simulink library "inp"  (R2021b)
settings: Solver=VariableStepAuto  StartTime=0.0  StopTime=10.0  RelTol=1e-3
undefined symbols (not defined in the file): C_TASK_5MS_S, FALSE, KINP_AcoreReadyToSlp_flg_ovrdflg, KINP_AcoreReadyToSlp_flg_ovrdval, KINP_AllowMovThd_OTA_enum_ovrdflg, KINP_AllowMovThd_OTA_enum_ovrdval, KINP_APSAngleTarget_Deg_ovrdflg, KINP_APSAngleTarget_Deg_ovrdval, KINP_APSDecReq_mps2_ovrdflg, KINP_APSDecReq_mps2_ovrdval, KINP_APSDecReqA_flg_ovrdflg, KINP_APSDecReqA_flg_ovrdval, KINP_APSDFLL_cm_ovrdflg, KINP_APSDFLL_cm_ovrdval, KINP_APSDFLR_cm_ovrdflg, KINP_APSDFLR_cm_ovrdval, KINP_APSDRLL_cm_ovrdflg, KINP_APSDRLL_cm_ovrdval, KINP_APSDRLR_cm_ovrdflg, KINP_APSDRLR_cm_ovrdval, KINP_APSExitCondition_enum_ovrdflg, KINP_APSExitCondition_enum_ovrdval, KINP_APSHWVer_enum_ovrdflg, KINP_APSHWVer_enum_ovrdval, KINP_APSProgressPCT_pct_ovrdflg, KINP_APSProgressPCT_pct_ovrdval, KINP_APSPwrReq_enum_ovrdflg, KINP_APSPwrReq_enum_ovrdval, KINP_APSReq_enum_ovrdflg, KINP_APSReq_enum_ovrdval, KINP_APSRQDisplay_enum_ovrdflg, KINP_APSRQDisplay_enum_ovrdval, KINP_APSRqEPASCtrl_flg_ovrdflg, KINP_APSRqEPASCtrl_flg_ovrdval, KINP_APSShiftPosnReq_enum_ovrdval, KINP_APSShiftPosnReq_enum_ovrflg, KINP_APSSpeedCMD_kph_ovrdval, KINP_APSSpeedCMD_kph_ovrflg, KINP_APSStaSystem_enum_ovrdflg, KINP_APSStaSystem_enum_ovrdval, KINP_APSSWVer_enum_ovrdflg, KINP_APSSWVer_enum_ovrdval, KINP_APSVMCReqA_flg_ovrdval, KINP_APSVMCReqA_flg_ovrflg, KINP_APSVRqEPASCtrl_flg_ovrdflg, KINP_APSVRqEPASCtrl_flg_ovrdval, KINP_AuxBattVolmV_mV_ovrdflg, KINP_AuxBattVolmV_mV_ovrdval, KINP_CAASSta_enum_ovrdflg, KINP_CAASSta_enum_ovrdval, KINP_CAASVMCReqA_flg_ovrdval, KINP_CAASVMCReqA_flg_ovrflg, KINP_CAN1BusOff_flg_ovrdflg, KINP_CAN1BusOff_flg_ovrdval, KINP_CAN2BusOff_flg_ovrdflg, KINP_CAN2BusOff_flg_ovrdval, KINP_CAN3BusOff_flg_ovrdflg, KINP_CAN3BusOff_flg_ovrdval, KINP_CAN4BusOff_flg_ovrdflg, KINP_CAN4BusOff_flg_ovrdval ... (+152)
libraries: FVT_lib x1037, hcu_lib x1
(part 6 of 34)

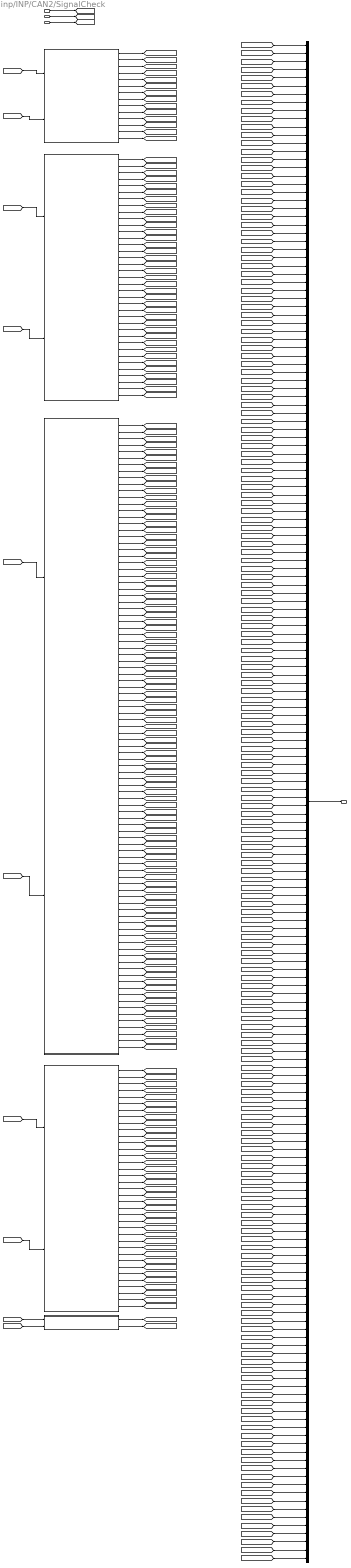
== system inp/INP/CAN2/SignalCheck ==
  inp_CanValid_bus : Inport
  TASK_TIME_S : Inport  Port=2
  BHAL_outputs : Inport  Port=3
  HMI1 : Subsystem
  IVI1 : Subsystem
  IVI2 : Subsystem
  IVI3 : Subsystem
  METER1 : Subsystem
  bus_creator : BusCreator  Inputs=186
  inp_Hal_bus : Outport
  wires:
  inp_CanValid_bus/1 -> [inp_CanValid_bus]
  TASK_TIME_S/1 -> [TASK_TIME_S]
  BHAL_outputs/1 -> [BHAL_outputs]
  [BHAL_outputs] -> HMI1/1(BHAL_outputs)
  [inp_CanValid_bus] -> HMI1/2(inp_CanValid_bus)
  HMI1/1(VINP_HMIACAirIntMCmd_flg) -> [VINP_HMIACAirIntMCmd_flg]
  HMI1/2(VINP_HMIACAirIntPCmd_flg) -> [VINP_HMIACAirIntPCmd_flg]
  HMI1/3(VINP_HMIACAutoBtnCmd_flg) -> [VINP_HMIACAutoBtnCmd_flg]
  HMI1/4(VINP_HMIACBtnCmd_flg) -> [VINP_HMIACBtnCmd_flg]
  HMI1/5(VINP_HMIACFrDefogBtnCmd_flg) -> [VINP_HMIACFrDefogBtnCmd_flg]
  HMI1/6(VINP_HMIACRecycleBtnCmd_flg) -> [VINP_HMIACRecycleBtnCmd_flg]
  HMI1/7(VINP_HMIACWindDirMCmd_flg) -> [VINP_HMIACWindDirMCmd_flg]
  HMI1/8(VINP_HMIACWindDirPCmd_flg) -> [VINP_HMIACWindDirPCmd_flg]
  HMI1/9(VINP_HMIAutoInterLightCmd_flg) -> [VINP_HMIAutoInterLightCmd_flg]
  HMI1/10(VINP_HMIBCMPostDefogBtnCmd_flg) -> [VINP_HMIBCMPostDefogBtnCmd_flg]
  HMI1/11(VINP_HMIZ1SetTMCmd_flg) -> [VINP_HMIZ1SetTMCmd_flg]
  HMI1/12(VINP_HMIZ1SetTPCmd_flg) -> [VINP_HMIZ1SetTPCmd_flg]
  HMI1/13(VINP_HMIZ2SetTMCmd_flg) -> [VINP_HMIZ2SetTMCmd_flg]
  HMI1/14(VINP_HMIZ2SetTPCmd_flg) -> [VINP_HMIZ2SetTPCmd_flg]
  [BHAL_outputs] -> IVI1/1(BHAL_outputs)
  [inp_CanValid_bus] -> IVI1/2(inp_CanValid_bus)
  IVI1/1(VINP_AmbLighLowBatAlertSW_flg) -> [VINP_AmbLighLowBatAlertSW_flg]
  IVI1/2(VINP_AmbLighSafetyAlertSW_flg) -> [VINP_AmbLighSafetyAlertSW_flg]
  IVI1/3(VINP_AmbLightBrightnessSet_enum) -> [VINP_AmbLightBrightnessSet_enum]
  IVI1/4(VINP_AmbLightColorSet_enum) -> [VINP_AmbLightColorSet_enum]
  IVI1/5(VINP_AmbLightDimInDarkSW_flg) -> [VINP_AmbLightDimInDarkSW_flg]
  IVI1/6(VINP_AmbLightSW_flg) -> [VINP_AmbLightSW_flg]
  IVI1/7(VINP_AmbLightWlcmLightSW_flg) -> [VINP_AmbLightWlcmLightSW_flg]
  IVI1/8(VINP_FCPFrEvtBtnACMaxReq_flg) -> [VINP_FCPFrEvtBtnACMaxReq_flg]
  IVI1/9(VINP_FCPFrEvtBtnACReq_flg) -> [VINP_FCPFrEvtBtnACReq_flg]
  IVI1/10(VINP_FCPFrEvtBtnAutoReq_flg) -> [VINP_FCPFrEvtBtnAutoReq_flg]
  IVI1/11(VINP_FCPFrEvtBtnSyncReq_flg) -> [VINP_FCPFrEvtBtnSyncReq_flg]
  IVI1/12(VINP_IVIAutoWipHSpdSWCmd_flg) -> [VINP_IVIAutoWipHSpdSWCmd_flg]
  IVI1/13(VINP_IVICreateAccReqSta_enum) -> [VINP_IVICreateAccReqSta_enum]
  IVI1/14(VINP_IVIDelAccReqSta_enum) -> [VINP_IVIDelAccReqSta_enum]
  IVI1/15(VINP_IVIDrivingLockSWSta_flg) -> [VINP_IVIDrivingLockSWSta_flg]
  IVI1/16(VINP_IVIFrTrunkUnlockReqSta_flg) -> [VINP_IVIFrTrunkUnlockReqSta_flg]
  IVI1/17(VINP_IVILinkAccReqSta_flg) -> [VINP_IVILinkAccReqSta_flg]
  IVI1/18(VINP_IVILinkAccSta_enum) -> [VINP_IVILinkAccSta_enum]
  IVI1/19(VINP_IVILinkKeySta_enum) -> [VINP_IVILinkKeySta_enum]
  IVI1/20(VINP_IVILocatedSTA_enum) -> [VINP_IVILocatedSTA_enum]
  IVI1/21(VINP_IVILockSoundSWSta_flg) -> [VINP_IVILockSoundSWSta_flg]
  IVI1/22(VINP_IVISWCVibModeSta_enum) -> [VINP_IVISWCVibModeSta_enum]
  IVI1/23(VINP_IVIStoppingUnlockSWSta_flg) -> [VINP_IVIStoppingUnlockSWSta_flg]
  IVI1/24(VINP_IVITimeCheck_enum) -> [VINP_IVITimeCheck_enum]
  IVI1/25(VINP_IVITimeDay_DAY) -> [VINP_IVITimeDay_DAY]
  IVI1/26(VINP_IVITimeHour_hr) -> [VINP_IVITimeHour_hr]
  IVI1/27(VINP_IVITimeMinute_min) -> [VINP_IVITimeMinute_min]
  IVI1/28(VINP_IVITimeMonth_MONTH) -> [VINP_IVITimeMonth_MONTH]
  IVI1/29(VINP_IVITimeSecond_s) -> [VINP_IVITimeSecond_s]
  IVI1/30(VINP_IVITimeYear_YEAR) -> [VINP_IVITimeYear_YEAR]
  IVI1/31(VINP_IVIWPTCSWSta_flg) -> [VINP_IVIWPTCSWSta_flg]
  IVI1/32(VINP_IVIsigScreenReqSta_flg) -> [VINP_IVIsigScreenReqSta_flg]
  IVI1/33(VINP_LINKtoDrive_flg) -> [VINP_LINKtoDrive_flg]
  IVI1/34(VINP_OpenDrOpenWdoSW_flg) -> [VINP_OpenDrOpenWdoSW_flg]
  IVI1/35(VINP_PWCONTINUEUSE_flg) -> [VINP_PWCONTINUEUSE_flg]
  IVI1/36(VINP_SmartEcoModeSW_flg) -> [VINP_SmartEcoModeSW_flg]
  IVI1/37(VINP_UserSet_enum) -> [VINP_UserSet_enum]
  [BHAL_outputs] -> IVI2/1(BHAL_outputs)
  [inp_CanValid_bus] -> IVI2/2(inp_CanValid_bus)
  IVI2/1(VINP_ACChgCurSet_A) -> [VINP_ACChgCurSet_A]
  IVI2/2(VINP_AVMErrSTA_flg) -> [VINP_AVMErrSTA_flg]
  IVI2/3(VINP_AVMOFFRecButt_flg) -> [VINP_AVMOFFRecButt_flg]
  IVI2/4(VINP_AVMParkingmode_enum) -> [VINP_AVMParkingmode_enum]
  IVI2/5(VINP_AVMparkingcancel_enum) -> [VINP_AVMparkingcancel_enum]
  IVI2/6(VINP_AVMparkingexcute_enum) -> [VINP_AVMparkingexcute_enum]
  IVI2/7(VINP_ApproachUnlockSW_flg) -> [VINP_ApproachUnlockSW_flg]
  IVI2/8(VINP_CAASSw_enum) -> [VINP_CAASSw_enum]
  IVI2/9(VINP_CDLLockButt_flg) -> [VINP_CDLLockButt_flg]
  IVI2/10(VINP_CDLUnlockButt_flg) -> [VINP_CDLUnlockButt_flg]
  IVI2/11(VINP_DSEATantiset_flg) -> [VINP_DSEATantiset_flg]
  IVI2/12(VINP_DSEATentryfunset_flg) -> [VINP_DSEATentryfunset_flg]
  IVI2/13(VINP_DSEATventreq_enum) -> [VINP_DSEATventreq_enum]
  IVI2/14(VINP_Distanceunit_flg) -> [VINP_Distanceunit_flg]
  IVI2/15(VINP_ESCSWCmd_enum) -> [VINP_ESCSWCmd_enum]
  IVI2/16(VINP_FSOffSw_enum) -> [VINP_FSOffSw_enum]
  IVI2/17(VINP_FollowMeSW_flg) -> [VINP_FollowMeSW_flg]
  IVI2/18(VINP_GPSLAT_s) -> [VINP_GPSLAT_s]
  IVI2/19(VINP_GPSLONG_enum) -> [VINP_GPSLONG_enum]
  IVI2/20(VINP_HeadLampSW_enum) -> [VINP_HeadLampSW_enum]
  IVI2/21(VINP_HoodLatchSW_enum) -> [VINP_HoodLatchSW_enum]
  IVI2/22(VINP_IVIACCAdaptiveSta_flg) -> [VINP_IVIACCAdaptiveSta_flg]
  IVI2/23(VINP_IVIAirIntZ3Cmd_enum) -> [VINP_IVIAirIntZ3Cmd_enum]
  IVI2/24(VINP_IVIChargePortSWSta_flg) -> [VINP_IVIChargePortSWSta_flg]
  IVI2/25(VINP_IVICreepSWReq_flg) -> [VINP_IVICreepSWReq_flg]
  IVI2/26(VINP_IVIDSEATHeaterCmd_enum) -> [VINP_IVIDSEATHeaterCmd_enum]
  IVI2/27(VINP_IVIDSEATFroEdgeHeightCmd_enum) -> [VINP_IVIDSEATFroEdgeHeightCmd_enum]
  IVI2/28(VINP_IVIDSEATHeightCmd_enum) -> [VINP_IVIDSEATHeightCmd_enum]
  IVI2/29(VINP_IVIDSEATMemory1Sta_flg) -> [VINP_IVIDSEATMemory1Sta_flg]
  IVI2/30(VINP_IVIDSEATMemory2Sta_flg) -> [VINP_IVIDSEATMemory2Sta_flg]
  IVI2/31(VINP_IVIDSEATMemoryOPTCLSSta_flg) -> [VINP_IVIDSEATMemoryOPTCLSSta_flg]
  IVI2/32(VINP_IVIDSEATReclineCmd_enum) -> [VINP_IVIDSEATReclineCmd_enum]
  IVI2/33(VINP_IVIDSEATSlideCmd_enum) -> [VINP_IVIDSEATSlideCmd_enum]
  IVI2/34(VINP_IVIFGSAirIntCmd_enum) -> [VINP_IVIFGSAirIntCmd_enum]
  IVI2/35(VINP_IVIFGSChCmd_enum) -> [VINP_IVIFGSChCmd_enum]
  IVI2/36(VINP_IVIIONSWCmd_flg) -> [VINP_IVIIONSWCmd_flg]
  IVI2/37(VINP_IVIISAOffsetSpd_enum) -> [VINP_IVIISAOffsetSpd_enum]
  IVI2/38(VINP_IVINightModeSta_flg) -> [VINP_IVINightModeSta_flg]
  IVI2/39(VINP_IVIPSEATHeaterCmd_enum) -> [VINP_IVIPSEATHeaterCmd_enum]
  IVI2/40(VINP_IVIPSEATReclineCmd_enum) -> [VINP_IVIPSEATReclineCmd_enum]
  IVI2/41(VINP_IVIPSEATSlideCmd_enum) -> [VINP_IVIPSEATSlideCmd_enum]
  IVI2/42(VINP_IVIPTGModeSW_enum) -> [VINP_IVIPTGModeSW_enum]
  IVI2/43(VINP_IVIPTGOpenHeight_enum) -> [VINP_IVIPTGOpenHeight_enum]
  IVI2/44(VINP_IVIPTGStaSW_enum) -> [VINP_IVIPTGStaSW_enum]
  IVI2/45(VINP_IVIPTGUSStaSW_flg) -> [VINP_IVIPTGUSStaSW_flg]
  IVI2/46(VINP_IVIPWModeReq_enum) -> [VINP_IVIPWModeReq_enum]
  IVI2/47(VINP_IVIPwrLockSW_enum) -> [VINP_IVIPwrLockSW_enum]
  IVI2/48(VINP_IVIPwroffreq_flg) -> [VINP_IVIPwroffreq_flg]
  IVI2/49(VINP_IVIRRDefReq_flg) -> [VINP_IVIRRDefReq_flg]
  IVI2/50(VINP_IVIReqV2L_enum) -> [VINP_IVIReqV2L_enum]
  IVI2/51(VINP_IVISWCRUndefinedSta_enum) -> [VINP_IVISWCRUndefinedSta_enum]
  IVI2/52(VINP_IVIScreen_enum) -> [VINP_IVIScreen_enum]
  IVI2/53(VINP_IVIStartChgreq_flg) -> [VINP_IVIStartChgreq_flg]
  IVI2/54(VINP_IVIStatus_flg) -> [VINP_IVIStatus_flg]
  IVI2/55(VINP_IVIStopChgreq_flg) -> [VINP_IVIStopChgreq_flg]
  IVI2/56(VINP_IVITrailerCheckReqSta_flg) -> [VINP_IVITrailerCheckReqSta_flg]
  IVI2/57(VINP_IVITrailerModeSWSta_flg) -> [VINP_IVITrailerModeSWSta_flg]
  IVI2/58(VINP_IVITriggerreq_flg) -> [VINP_IVITriggerreq_flg]
  IVI2/59(VINP_IVIUnlockChgreq_flg) -> [VINP_IVIUnlockChgreq_flg]
  IVI2/60(VINP_IVIWIMAINSW_flg) -> [VINP_IVIWIMAINSW_flg]
  IVI2/61(VINP_LDrvControlCommand_pct) -> [VINP_LDrvControlCommand_pct]
  IVI2/62(VINP_LPasControlCommand_pct) -> [VINP_LPasControlCommand_pct]
  IVI2/63(VINP_LRLDControlCommand_pct) -> [VINP_LRLDControlCommand_pct]
  IVI2/64(VINP_LRRDControlCommand_pct) -> [VINP_LRRDControlCommand_pct]
  IVI2/65(VINP_LightShowStartReq_flg) -> [VINP_LightShowStartReq_flg]
  IVI2/66(VINP_LightShowStopReq_flg) -> [VINP_LightShowStopReq_flg]
  IVI2/67(VINP_MFRDNBrightReq_pct) -> [VINP_MFRDNBrightReq_pct]
  IVI2/68(VINP_OFFACMODE_enum) -> [VINP_OFFACMODE_enum]
  IVI2/69(VINP_PSEATventreq_enum) -> [VINP_PSEATventreq_enum]
  IVI2/70(VINP_PerdV2L_enum) -> [VINP_PerdV2L_enum]
  IVI2/71(VINP_RFogLampSW_flg) -> [VINP_RFogLampSW_flg]
  IVI2/72(VINP_RollModeSWCmd_enum) -> [VINP_RollModeSWCmd_enum]
  IVI2/73(VINP_RoomLampMode_flg) -> [VINP_RoomLampMode_flg]
  IVI2/74(VINP_SOCADJBUTT_flg) -> [VINP_SOCADJBUTT_flg]
  IVI2/75(VINP_SOCLimitSet_pct) -> [VINP_SOCLimitSet_pct]
  IVI2/76(VINP_SOCV2LLimit_pct) -> [VINP_SOCV2LLimit_pct]
  IVI2/77(VINP_SchedChgStart_flg) -> [VINP_SchedChgStart_flg]
  IVI2/78(VINP_SchedChgStop_flg) -> [VINP_SchedChgStop_flg]
  IVI2/79(VINP_SchedChgbutt_flg) -> [VINP_SchedChgbutt_flg]
  IVI2/80(VINP_SchedChglimit_pct) -> [VINP_SchedChglimit_pct]
  IVI2/81(VINP_SchedChgwake_flg) -> [VINP_SchedChgwake_flg]
  IVI2/82(VINP_SenstivityPosition_enum) -> [VINP_SenstivityPosition_enum]
  IVI2/83(VINP_SetUnlockSingle_flg) -> [VINP_SetUnlockSingle_flg]
  IVI2/84(VINP_TCSSWCmd_enum) -> [VINP_TCSSWCmd_enum]
  IVI2/85(VINP_TPMSCaliButt_flg) -> [VINP_TPMSCaliButt_flg]
  IVI2/86(VINP_TPMSResButt_flg) -> [VINP_TPMSResButt_flg]
  IVI2/87(VINP_TurnSwTimeSet_enum) -> [VINP_TurnSwTimeSet_enum]
  IVI2/88(VINP_WalkawayLockSW_flg) -> [VINP_WalkawayLockSW_flg]
  IVI2/89(VINP_WlcmLightMode_enum) -> [VINP_WlcmLightMode_enum]
  IVI2/90(VINP_sigAirIntenZon1Req_enum) -> [VINP_sigAirIntenZon1Req_enum]
  IVI2/91(VINP_sigDfrstReq_flg) -> [VINP_sigDfrstReq_flg]
  IVI2/92(VINP_sigFaceReq_flg) -> [VINP_sigFaceReq_flg]
  IVI2/93(VINP_sigFootReq_flg) -> [VINP_sigFootReq_flg]
  IVI2/94(VINP_sigRecircReq_flg) -> [VINP_sigRecircReq_flg]
  IVI2/95(VINP_sigSetTempZon1Req_C) -> [VINP_sigSetTempZon1Req_C]
  IVI2/96(VINP_sigSetTempZon2Req_C) -> [VINP_sigSetTempZon2Req_C]
  [BHAL_outputs] -> IVI3/1(BHAL_outputs)
  [inp_CanValid_bus] -> IVI3/2(inp_CanValid_bus)
  IVI3/1(VINP_IVICLBlowerYSta_pct) -> [VINP_IVICLBlowerYSta_pct]
  IVI3/2(VINP_IVICLBlowerZSta_pct) -> [VINP_IVICLBlowerZSta_pct]
  IVI3/3(VINP_IVICRBlowerYSta_pct) -> [VINP_IVICRBlowerYSta_pct]
  IVI3/4(VINP_IVICRBlowerZSta_pct) -> [VINP_IVICRBlowerZSta_pct]
  IVI3/5(VINP_IVIDrBlowerModeSta_enum) -> [VINP_IVIDrBlowerModeSta_enum]
  IVI3/6(VINP_IVIDrBlowerYSta_pct) -> [VINP_IVIDrBlowerYSta_pct]
  IVI3/7(VINP_IVIDrBlowerZSta_pct) -> [VINP_IVIDrBlowerZSta_pct]
  IVI3/8(VINP_IVIHMICustmiFunSta_enum) -> [VINP_IVIHMICustmiFunSta_enum]
  IVI3/9(VINP_IVIHMICustmiKEYSta_enum) -> [VINP_IVIHMICustmiKEYSta_enum]
  IVI3/10(VINP_IVILSEATventCmd_enum) -> [VINP_IVILSEATventCmd_enum]
  IVI3/11(VINP_IVIMLFMostCmd_flg) -> [VINP_IVIMLFMostCmd_flg]
  IVI3/12(VINP_IVIMLFootLiftCmd_enum) -> [VINP_IVIMLFootLiftCmd_enum]
  IVI3/13(VINP_IVIMLNapModeCmd_flg) -> [VINP_IVIMLNapModeCmd_flg]
  IVI3/14(VINP_IVIMLReclinerCmd_enum) -> [VINP_IVIMLReclinerCmd_enum]
  IVI3/15(VINP_IVIMLRestoreCmd_flg) -> [VINP_IVIMLRestoreCmd_flg]
  IVI3/16(VINP_IVIMLSEATventCmd_enum) -> [VINP_IVIMLSEATventCmd_enum]
  IVI3/17(VINP_IVIMLSeatLiftCmd_enum) -> [VINP_IVIMLSeatLiftCmd_enum]
  IVI3/18(VINP_IVIMLSldRestoreCmd_flg) -> [VINP_IVIMLSldRestoreCmd_flg]
  IVI3/19(VINP_IVIMLSliderCmd_enum) -> [VINP_IVIMLSliderCmd_enum]
  IVI3/20(VINP_IVIMLZeroGravityCmd_flg) -> [VINP_IVIMLZeroGravityCmd_flg]
  IVI3/21(VINP_IVIMRFMostCmd_flg) -> [VINP_IVIMRFMostCmd_flg]
  IVI3/22(VINP_IVIMRFootLiftCmd_enum) -> [VINP_IVIMRFootLiftCmd_enum]
  IVI3/23(VINP_IVIMRNapModeCmd_flg) -> [VINP_IVIMRNapModeCmd_flg]
  IVI3/24(VINP_IVIMRReclinerCmd_enum) -> [VINP_IVIMRReclinerCmd_enum]
  IVI3/25(VINP_IVIMRRestoreCmd_flg) -> [VINP_IVIMRRestoreCmd_flg]
  IVI3/26(VINP_IVIMRSEATventCmd_enum) -> [VINP_IVIMRSEATventCmd_enum]
  IVI3/27(VINP_IVIMRSeatLiftCmd_enum) -> [VINP_IVIMRSeatLiftCmd_enum]
  IVI3/28(VINP_IVIMRSldRestoreCmd_flg) -> [VINP_IVIMRSldRestoreCmd_flg]
  IVI3/29(VINP_IVIMRSliderCmd_enum) -> [VINP_IVIMRSliderCmd_enum]
  IVI3/30(VINP_IVIMRZeroGravityCmd_flg) -> [VINP_IVIMRZeroGravityCmd_flg]
  IVI3/31(VINP_IVIPsBlowerModeSta_enum) -> [VINP_IVIPsBlowerModeSta_enum]
  IVI3/32(VINP_IVIPsBlowerYSta_pct) -> [VINP_IVIPsBlowerYSta_pct]
  IVI3/33(VINP_IVIPsBlowerZSta_pct) -> [VINP_IVIPsBlowerZSta_pct]
  IVI3/34(VINP_IVIRSEATventCmd_enum) -> [VINP_IVIRSEATventCmd_enum]
  IVI3/35(VINP_IVISnowModeCmd_flg) -> [VINP_IVISnowModeCmd_flg]
  IVI3/36(VINP_IVIUserTakeOverAPSSta_flg) -> [VINP_IVIUserTakeOverAPSSta_flg]
  IVI3/37(VINP_IVIZon1WindDirSWReqSta_flg) -> [VINP_IVIZon1WindDirSWReqSta_flg]
  [BHAL_outputs] -> METER1/1(BHAL_outputs)
  [inp_CanValid_bus] -> METER1/2(inp_CanValid_bus)
  METER1/1(VINP_METERKPHCalcu_kph) -> [VINP_METERKPHCalcu_kph]
  METER1/2(VINP_ODOMETER_km) -> [VINP_ODOMETER_km]
  bus_creator/1 -> inp_Hal_bus/1
  [VINP_HMIACAirIntMCmd_flg] -> bus_creator/1
  [VINP_HMIACAirIntPCmd_flg] -> bus_creator/2
  [VINP_HMIACAutoBtnCmd_flg] -> bus_creator/3
  [VINP_HMIACBtnCmd_flg] -> bus_creator/4
  [VINP_HMIACFrDefogBtnCmd_flg] -> bus_creator/5
  [VINP_HMIACRecycleBtnCmd_flg] -> bus_creator/6
  [VINP_HMIACWindDirMCmd_flg] -> bus_creator/7
  [VINP_HMIACWindDirPCmd_flg] -> bus_creator/8
  [VINP_HMIAutoInterLightCmd_flg] -> bus_creator/9
  [VINP_HMIBCMPostDefogBtnCmd_flg] -> bus_creator/10
  [VINP_HMIZ1SetTMCmd_flg] -> bus_creator/11
  [VINP_HMIZ1SetTPCmd_flg] -> bus_creator/12
  [VINP_HMIZ2SetTMCmd_flg] -> bus_creator/13
  [VINP_HMIZ2SetTPCmd_flg] -> bus_creator/14
  [VINP_AmbLighLowBatAlertSW_flg] -> bus_creator/15
  [VINP_AmbLighSafetyAlertSW_flg] -> bus_creator/16
  [VINP_AmbLightBrightnessSet_enum] -> bus_creator/17
  [VINP_AmbLightColorSet_enum] -> bus_creator/18
  [VINP_AmbLightDimInDarkSW_flg] -> bus_creator/19
  [VINP_AmbLightSW_flg] -> bus_creator/20
  [VINP_AmbLightWlcmLightSW_flg] -> bus_creator/21
  [VINP_FCPFrEvtBtnACMaxReq_flg] -> bus_creator/22
  [VINP_FCPFrEvtBtnACReq_flg] -> bus_creator/23
  [VINP_FCPFrEvtBtnAutoReq_flg] -> bus_creator/24
  [VINP_FCPFrEvtBtnSyncReq_flg] -> bus_creator/25
  [VINP_IVIAutoWipHSpdSWCmd_flg] -> bus_creator/26
  [VINP_IVICreateAccReqSta_enum] -> bus_creator/27
  [VINP_IVIDelAccReqSta_enum] -> bus_creator/28
  [VINP_IVIDrivingLockSWSta_flg] -> bus_creator/29
  [VINP_IVIFrTrunkUnlockReqSta_flg] -> bus_creator/30
  [VINP_IVILinkAccReqSta_flg] -> bus_creator/31
  [VINP_IVILinkAccSta_enum] -> bus_creator/32
  [VINP_IVILinkKeySta_enum] -> bus_creator/33
  [VINP_IVILocatedSTA_enum] -> bus_creator/34
  [VINP_IVILockSoundSWSta_flg] -> bus_creator/35
  [VINP_IVISWCVibModeSta_enum] -> bus_creator/36
  [VINP_IVIStoppingUnlockSWSta_flg] -> bus_creator/37
  [VINP_IVITimeCheck_enum] -> bus_creator/38
  [VINP_IVITimeDay_DAY] -> bus_creator/39
  [VINP_IVITimeHour_hr] -> bus_creator/40
  [VINP_IVITimeMinute_min] -> bus_creator/41
  [VINP_IVITimeMonth_MONTH] -> bus_creator/42
  [VINP_IVITimeSecond_s] -> bus_creator/43
  [VINP_IVITimeYear_YEAR] -> bus_creator/44
  [VINP_IVIWPTCSWSta_flg] -> bus_creator/45
  [VINP_IVIsigScreenReqSta_flg] -> bus_creator/46
  [VINP_LINKtoDrive_flg] -> bus_creator/47
  [VINP_OpenDrOpenWdoSW_flg] -> bus_creator/48
  [VINP_PWCONTINUEUSE_flg] -> bus_creator/49
  [VINP_SmartEcoModeSW_flg] -> bus_creator/50
  [VINP_UserSet_enum] -> bus_creator/51
  [VINP_ACChgCurSet_A] -> bus_creator/52
  [VINP_AVMErrSTA_flg] -> bus_creator/53
  [VINP_AVMOFFRecButt_flg] -> bus_creator/54
  [VINP_AVMParkingmode_enum] -> bus_creator/55
  [VINP_AVMparkingcancel_enum] -> bus_creator/56
  [VINP_AVMparkingexcute_enum] -> bus_creator/57
  [VINP_ApproachUnlockSW_flg] -> bus_creator/58
  [VINP_CAASSw_enum] -> bus_creator/59
  [VINP_CDLLockButt_flg] -> bus_creator/60
  [VINP_CDLUnlockButt_flg] -> bus_creator/61
  [VINP_DSEATantiset_flg] -> bus_creator/62
  [VINP_DSEATentryfunset_flg] -> bus_creator/63
  [VINP_DSEATventreq_enum] -> bus_creator/64
  [VINP_Distanceunit_flg] -> bus_creator/65
  [VINP_ESCSWCmd_enum] -> bus_creator/66
  [VINP_FSOffSw_enum] -> bus_creator/67
  [VINP_FollowMeSW_flg] -> bus_creator/68
  [VINP_GPSLAT_s] -> bus_creator/69
  [VINP_GPSLONG_enum] -> bus_creator/70
  [VINP_HeadLampSW_enum] -> bus_creator/71
  [VINP_HoodLatchSW_enum] -> bus_creator/72
  [VINP_IVIACCAdaptiveSta_flg] -> bus_creator/73
  [VINP_IVIAirIntZ3Cmd_enum] -> bus_creator/74
  [VINP_IVIChargePortSWSta_flg] -> bus_creator/75
  [VINP_IVICreepSWReq_flg] -> bus_creator/76
  [VINP_IVIDSEATHeaterCmd_enum] -> bus_creator/77
  [VINP_IVIDSEATFroEdgeHeightCmd_enum] -> bus_creator/78
  [VINP_IVIDSEATHeightCmd_enum] -> bus_creator/79
  [VINP_IVIDSEATMemory1Sta_flg] -> bus_creator/80
  [VINP_IVIDSEATMemory2Sta_flg] -> bus_creator/81
  [VINP_IVIDSEATMemoryOPTCLSSta_flg] -> bus_creator/82
  [VINP_IVIDSEATReclineCmd_enum] -> bus_creator/83
  [VINP_IVIDSEATSlideCmd_enum] -> bus_creator/84
  [VINP_IVIFGSAirIntCmd_enum] -> bus_creator/85
  [VINP_IVIFGSChCmd_enum] -> bus_creator/86
  [VINP_IVIIONSWCmd_flg] -> bus_creator/87
  [VINP_IVIISAOffsetSpd_enum] -> bus_creator/88
  [VINP_IVINightModeSta_flg] -> bus_creator/89
  [VINP_IVIPSEATHeaterCmd_enum] -> bus_creator/90
  [VINP_IVIPSEATReclineCmd_enum] -> bus_creator/91
  [VINP_IVIPSEATSlideCmd_enum] -> bus_creator/92
  [VINP_IVIPTGModeSW_enum] -> bus_creator/93
  [VINP_IVIPTGOpenHeight_enum] -> bus_creator/94
  [VINP_IVIPTGStaSW_enum] -> bus_creator/95
  [VINP_IVIPTGUSStaSW_flg] -> bus_creator/96
  [VINP_IVIPWModeReq_enum] -> bus_creator/97
  [VINP_IVIPwrLockSW_enum] -> bus_creator/98
  [VINP_IVIPwroffreq_flg] -> bus_creator/99
  [VINP_IVIRRDefReq_flg] -> bus_creator/100
  [VINP_IVIReqV2L_enum] -> bus_creator/101
  [VINP_IVISWCRUndefinedSta_enum] -> bus_creator/102
  [VINP_IVIScreen_enum] -> bus_creator/103
  [VINP_IVIStartChgreq_flg] -> bus_creator/104
  [VINP_IVIStatus_flg] -> bus_creator/105
  [VINP_IVIStopChgreq_flg] -> bus_creator/106
  [VINP_IVITrailerCheckReqSta_flg] -> bus_creator/107
  [VINP_IVITrailerModeSWSta_flg] -> bus_creator/108
  [VINP_IVITriggerreq_flg] -> bus_creator/109
  [VINP_IVIUnlockChgreq_flg] -> bus_creator/110
  [VINP_IVIWIMAINSW_flg] -> bus_creator/111
  [VINP_LDrvControlCommand_pct] -> bus_creator/112
  [VINP_LPasControlCommand_pct] -> bus_creator/113
  [VINP_LRLDControlCommand_pct] -> bus_creator/114
  [VINP_LRRDControlCommand_pct] -> bus_creator/115
  [VINP_LightShowStartReq_flg] -> bus_creator/116
  [VINP_LightShowStopReq_flg] -> bus_creator/117
  [VINP_MFRDNBrightReq_pct] -> bus_creator/118
  [VINP_OFFACMODE_enum] -> bus_creator/119
  [VINP_PSEATventreq_enum] -> bus_creator/120
  [VINP_PerdV2L_enum] -> bus_creator/121
  [VINP_RFogLampSW_flg] -> bus_creator/122
  [VINP_RollModeSWCmd_enum] -> bus_creator/123
  [VINP_RoomLampMode_flg] -> bus_creator/124
  [VINP_SOCADJBUTT_flg] -> bus_creator/125
  [VINP_SOCLimitSet_pct] -> bus_creator/126
  [VINP_SOCV2LLimit_pct] -> bus_creator/127
  [VINP_SchedChgStart_flg] -> bus_creator/128
  [VINP_SchedChgStop_flg] -> bus_creator/129
  [VINP_SchedChgbutt_flg] -> bus_creator/130
  [VINP_SchedChglimit_pct] -> bus_creator/131
  [VINP_SchedChgwake_flg] -> bus_creator/132
  [VINP_SenstivityPosition_enum] -> bus_creator/133
  [VINP_SetUnlockSingle_flg] -> bus_creator/134
  [VINP_TCSSWCmd_enum] -> bus_creator/135
  [VINP_TPMSCaliButt_flg] -> bus_creator/136
  [VINP_TPMSResButt_flg] -> bus_creator/137
  [VINP_TurnSwTimeSet_enum] -> bus_creator/138
  [VINP_WalkawayLockSW_flg] -> bus_creator/139
  [VINP_WlcmLightMode_enum] -> bus_creator/140
  [VINP_sigAirIntenZon1Req_enum] -> bus_creator/141
  [VINP_sigDfrstReq_flg] -> bus_creator/142
  [VINP_sigFaceReq_flg] -> bus_creator/143
  [VINP_sigFootReq_flg] -> bus_creator/144
  [VINP_sigRecircReq_flg] -> bus_creator/145
  [VINP_sigSetTempZon1Req_C] -> bus_creator/146
  [VINP_sigSetTempZon2Req_C] -> bus_creator/147
  [VINP_IVICLBlowerYSta_pct] -> bus_creator/148
  [VINP_IVICLBlowerZSta_pct] -> bus_creator/149
  [VINP_IVICRBlowerYSta_pct] -> bus_creator/150
  [VINP_IVICRBlowerZSta_pct] -> bus_creator/151
  [VINP_IVIDrBlowerModeSta_enum] -> bus_creator/152
  [VINP_IVIDrBlowerYSta_pct] -> bus_creator/153
  [VINP_IVIDrBlowerZSta_pct] -> bus_creator/154
  [VINP_IVIHMICustmiFunSta_enum] -> bus_creator/155
  [VINP_IVIHMICustmiKEYSta_enum] -> bus_creator/156
  [VINP_IVILSEATventCmd_enum] -> bus_creator/157
  [VINP_IVIMLFMostCmd_flg] -> bus_creator/158
  [VINP_IVIMLFootLiftCmd_enum] -> bus_creator/159
  [VINP_IVIMLNapModeCmd_flg] -> bus_creator/160
  [VINP_IVIMLReclinerCmd_enum] -> bus_creator/161
  [VINP_IVIMLRestoreCmd_flg] -> bus_creator/162
  [VINP_IVIMLSEATventCmd_enum] -> bus_creator/163
  [VINP_IVIMLSeatLiftCmd_enum] -> bus_creator/164
  [VINP_IVIMLSldRestoreCmd_flg] -> bus_creator/165
  [VINP_IVIMLSliderCmd_enum] -> bus_creator/166
  [VINP_IVIMLZeroGravityCmd_flg] -> bus_creator/167
  [VINP_IVIMRFMostCmd_flg] -> bus_creator/168
  [VINP_IVIMRFootLiftCmd_enum] -> bus_creator/169
  [VINP_IVIMRNapModeCmd_flg] -> bus_creator/170
  [VINP_IVIMRReclinerCmd_enum] -> bus_creator/171
  [VINP_IVIMRRestoreCmd_flg] -> bus_creator/172
  [VINP_IVIMRSEATventCmd_enum] -> bus_creator/173
  [VINP_IVIMRSeatLiftCmd_enum] -> bus_creator/174
  [VINP_IVIMRSldRestoreCmd_flg] -> bus_creator/175
  [VINP_IVIMRSliderCmd_enum] -> bus_creator/176
  [VINP_IVIMRZeroGravityCmd_flg] -> bus_creator/177
  [VINP_IVIPsBlowerModeSta_enum] -> bus_creator/178
  [VINP_IVIPsBlowerYSta_pct] -> bus_creator/179
  [VINP_IVIPsBlowerZSta_pct] -> bus_creator/180
  [VINP_IVIRSEATventCmd_enum] -> bus_creator/181
  [VINP_IVISnowModeCmd_flg] -> bus_creator/182
  [VINP_IVIUserTakeOverAPSSta_flg] -> bus_creator/183
  [VINP_IVIZon1WindDirSWReqSta_flg] -> bus_creator/184
  [VINP_METERKPHCalcu_kph] -> bus_creator/185
  [VINP_ODOMETER_km] -> bus_creator/186

== system inp/INP/CAN3/CommunicationCheck ==
  BHAL_outputs : Inport
  CANMsgInvalidBMS1 : FVT_lib/inp/CAN_Msg_Validity_Process_template  SystemSampleTime=-1  VariantActivationTime=update diagram  Latency=0  AutoFrameSizeCalculation=off
      link override ovrdflg: Value=KINP_CANMsgInvalidBMS1_flg_ovrdflg
      link override ovrdval: Value=KINP_CANMsgInvalidBMS1_flg_ovrdval
  CANMsgInvalidBMS3 : FVT_lib/inp/CAN_Msg_Validity_Process_template  SystemSampleTime=-1  VariantActivationTime=update diagram  Latency=0  AutoFrameSizeCalculation=off
      link override ovrdflg: Value=KINP_CANMsgInvalidBMS3_flg_ovrdflg
      link override ovrdval: Value=KINP_CANMsgInvalidBMS3_flg_ovrdval
  CANMsgInvalidBMS4 : FVT_lib/inp/CAN_Msg_Validity_Process_template  SystemSampleTime=-1  VariantActivationTime=update diagram  Latency=0  AutoFrameSizeCalculation=off
      link override ovrdflg: Value=KINP_CANMsgInvalidBMS4_flg_ovrdflg
      link override ovrdval: Value=KINP_CANMsgInvalidBMS4_flg_ovrdval
  CANMsgInvalidBMS5 : FVT_lib/inp/CAN_Msg_Validity_Process_template  SystemSampleTime=-1  VariantActivationTime=update diagram  Latency=0  AutoFrameSizeCalculation=off
      link override ovrdflg: Value=KINP_CANMsgInvalidBMS5_flg_ovrdflg
      link override ovrdval: Value=KINP_CANMsgInvalidBMS5_flg_ovrdval
  CANMsgInvalidBMS6 : FVT_lib/inp/CAN_Msg_Validity_Process_template  SystemSampleTime=-1  VariantActivationTime=update diagram  Latency=0  AutoFrameSizeCalculation=off
      link override ovrdflg: Value=KINP_CANMsgInvalidBMS6_flg_ovrdflg
      link override ovrdval: Value=KINP_CANMsgInvalidBMS6_flg_ovrdval
  CANMsgInvalidBMS8 : FVT_lib/inp/CAN_Msg_Validity_Process_template  SystemSampleTime=-1  VariantActivationTime=update diagram  Latency=0  AutoFrameSizeCalculation=off
      link override ovrdflg: Value=KINP_CANMsgInvalidBMS8_flg_ovrdflg
      link override ovrdval: Value=KINP_CANMsgInvalidBMS8_flg_ovrdval
  CANMsgInvalidCCU1 : FVT_lib/inp/CAN_Msg_Validity_Process_template  SystemSampleTime=-1  VariantActivationTime=update diagram  Latency=0  AutoFrameSizeCalculation=off
      link override ovrdflg: Value=KINP_CANMsgInvalidCCU1_flg_ovrdflg
      link override ovrdval: Value=KINP_CANMsgInvalidCCU1_flg_ovrdval
  CANMsgInvalidCCU2 : FVT_lib/inp/CAN_Msg_Validity_Process_template  SystemSampleTime=-1  VariantActivationTime=update diagram  Latency=0  AutoFrameSizeCalculation=off
      link override ovrdflg: Value=KINP_CANMsgInvalidCCU2_flg_ovrdflg
      link override ovrdval: Value=KINP_CANMsgInvalidCCU2_flg_ovrdval
  CANMsgInvalidEBM1 : FVT_lib/inp/CAN_Msg_Validity_Process_template  SystemSampleTime=-1  VariantActivationTime=update diagram  Latency=0  AutoFrameSizeCalculation=off
      link override ovrdflg: Value=KINP_CANMsgInvalidEBM1_flg_ovrdflg
      link override ovrdval: Value=KINP_CANMsgInvalidEBM1_flg_ovrdval
  CANMsgInvalidMCUBF1 : FVT_lib/inp/CAN_Msg_Validity_Process_template  SystemSampleTime=-1  VariantActivationTime=update diagram  Latency=0  AutoFrameSizeCalculation=off
      link override ovrdflg: Value=KINP_CANMsgInvalidMCUBF1_flg_ovrdflg
      link override ovrdval: Value=KINP_CANMsgInvalidMCUBF1_flg_ovrdval
  CANMsgInvalidMCUBF2 : FVT_lib/inp/CAN_Msg_Validity_Process_template  SystemSampleTime=-1  VariantActivationTime=update diagram  Latency=0  AutoFrameSizeCalculation=off
      link override ovrdflg: Value=KINP_CANMsgInvalidMCUBF2_flg_ovrdflg
      link override ovrdval: Value=KINP_CANMsgInvalidMCUBF2_flg_ovrdval
  CANMsgInvalidMCUBR1 : FVT_lib/inp/CAN_Msg_Validity_Process_template  SystemSampleTime=-1  VariantActivationTime=update diagram  Latency=0  AutoFrameSizeCalculation=off
      link override ovrdflg: Value=KINP_CANMsgInvalidMCUBR1_flg_ovrdflg
      link override ovrdval: Value=KINP_CANMsgInvalidMCUBR1_flg_ovrdval
  CANMsgInvalidMCUBR2 : FVT_lib/inp/CAN_Msg_Validity_Process_template  SystemSampleTime=-1  VariantActivationTime=update diagram  Latency=0  AutoFrameSizeCalculation=off
      link override ovrdflg: Value=KINP_CANMsgInvalidMCUBR2_flg_ovrdflg
      link override ovrdval: Value=KINP_CANMsgInvalidMCUBR2_flg_ovrdval
  CANMsgInvalidMCUNF1 : FVT_lib/inp/CAN_Msg_Validity_Process_template  SystemSampleTime=-1  VariantActivationTime=update diagram  Latency=0  AutoFrameSizeCalculation=off
      link override ovrdflg: Value=KINP_CANMsgInvalidMCUNF1_flg_ovrdflg
      link override ovrdval: Value=KINP_CANMsgInvalidMCUNF1_flg_ovrdval
  CANMsgInvalidMCUNF2 : FVT_lib/inp/CAN_Msg_Validity_Process_template  SystemSampleTime=-1  VariantActivationTime=update diagram  Latency=0  AutoFrameSizeCalculation=off
      link override ovrdflg: Value=KINP_CANMsgInvalidMCUNF2_flg_ovrdflg
      link override ovrdval: Value=KINP_CANMsgInvalidMCUNF2_flg_ovrdval
  CANMsgInvalidMCUNF3 : FVT_lib/inp/CAN_Msg_Validity_Process_template  SystemSampleTime=-1  VariantActivationTime=update diagram  Latency=0  AutoFrameSizeCalculation=off
      link override ovrdflg: Value=KINP_CANMsgInvalidMCUNF3_flg_ovrdflg
      link override ovrdval: Value=KINP_CANMsgInvalidMCUNF3_flg_ovrdval
  CANMsgInvalidMCUNR1 : FVT_lib/inp/CAN_Msg_Validity_Process_template  SystemSampleTime=-1  VariantActivationTime=update diagram  Latency=0  AutoFrameSizeCalculation=off
      link override ovrdflg: Value=KINP_CANMsgInvalidMCUNR1_flg_ovrdflg
      link override ovrdval: Value=KINP_CANMsgInvalidMCUNR1_flg_ovrdval
  CANMsgInvalidMCUNR2 : FVT_lib/inp/CAN_Msg_Validity_Process_template  SystemSampleTime=-1  VariantActivationTime=update diagram  Latency=0  AutoFrameSizeCalculation=off
      link override ovrdflg: Value=KINP_CANMsgInvalidMCUNR2_flg_ovrdflg
      link override ovrdval: Value=KINP_CANMsgInvalidMCUNR2_flg_ovrdval
  CANMsgInvalidMCUNR3 : FVT_lib/inp/CAN_Msg_Validity_Process_template  SystemSampleTime=-1  VariantActivationTime=update diagram  Latency=0  AutoFrameSizeCalculation=off
      link override ovrdflg: Value=KINP_CANMsgInvalidMCUNR3_flg_ovrdflg
      link override ovrdval: Value=KINP_CANMsgInvalidMCUNR3_flg_ovrdval
  CANMsgInvalidShifter1 : FVT_lib/inp/CAN_Msg_Validity_Process_template  SystemSampleTime=-1  VariantActivationTime=update diagram  Latency=0  AutoFrameSizeCalculation=off
      link override ovrdflg: Value=KINP_CANMsgInvalidShifter1_flg_ovrdflg
      link override ovrdval: Value=KINP_CANMsgInvalidShifter1_flg_ovrdval
  CANMsgInvalidShifter2 : FVT_lib/inp/CAN_Msg_Validity_Process_template  SystemSampleTime=-1  VariantActivationTime=update diagram  Latency=0  AutoFrameSizeCalculation=off
      link override ovrdflg: Value=KINP_CANMsgInvalidShifter2_flg_ovrdflg
      link override ovrdval: Value=KINP_CANMsgInvalidShifter2_flg_ovrdval
  bus_creator : BusCreator  Inputs=21
  bus_selector : BusSelector  OutputSignals=VHAL_CANMsgInvalidBMS1_flg,VHAL_CANMsgInvalidBMS3_flg,VHAL_CANMsgInvalidBMS4_flg,VHAL_CANMsgInvalidBMS5_flg,VHAL_CANMsgInvalidBMS6_flg,VHAL_CANMsgInvalidBMS8_flg,VHAL_CANMsgInvalidCCU1_flg,VHAL_CANMsgInvalidCCU2_flg,VHAL_CANMsgInvalidEBM1_flg,VHAL_CANMsgInvalidMCUBF1_flg,VHAL_CANMsgInvalidMCUBF2_flg,VHAL_CANMsgInvalidMCUBR1_flg,VHAL_CANMsgInvalidMCUBR2_flg,VHAL_CANMsgInvalidMCUNF1_flg,VHAL_CANMsgInvalidMCUNF2_flg,VHAL_CANMsgInvalidMCUNF3_flg,VHAL_CANMsgInvalidMCUNR1_flg,VHAL_CANMsgInvalidMCUNR2_flg,VHAL_CANMsgInvalidMCUNR3_flg,VHAL_CANMsgInvalidShifter1_flg,VHAL_CANMsgInvalidShifter2_flg
  not{1..21} (21 alike) : Logic  Operator=NOT  AllPortsSameDT=off  OutDataTypeStr=boolean
  inp_CanValid_bus : Outport
  wires:
  BHAL_outputs/1 -> [BHAL_outputs]
  bus_selector/1 -> CANMsgInvalidBMS1/1  "<VHAL_CANMsgInvalidBMS1_flg>"
  CANMsgInvalidBMS1/1 -> not1/1
  not1/1 -> bus_creator/1  "VINP_CANMsgValidBMS1_flg"
  bus_selector/2 -> CANMsgInvalidBMS3/1  "<VHAL_CANMsgInvalidBMS3_flg>"
  CANMsgInvalidBMS3/1 -> not2/1
  not2/1 -> bus_creator/2  "VINP_CANMsgValidBMS3_flg"
  bus_selector/3 -> CANMsgInvalidBMS4/1  "<VHAL_CANMsgInvalidBMS4_flg>"
  CANMsgInvalidBMS4/1 -> not3/1
  not3/1 -> bus_creator/3  "VINP_CANMsgValidBMS4_flg"
  bus_selector/4 -> CANMsgInvalidBMS5/1  "<VHAL_CANMsgInvalidBMS5_flg>"
  CANMsgInvalidBMS5/1 -> not4/1
  not4/1 -> bus_creator/4  "VINP_CANMsgValidBMS5_flg"
  bus_selector/5 -> CANMsgInvalidBMS6/1  "<VHAL_CANMsgInvalidBMS6_flg>"
  CANMsgInvalidBMS6/1 -> not5/1
  not5/1 -> bus_creator/5  "VINP_CANMsgValidBMS6_flg"
  bus_selector/6 -> CANMsgInvalidBMS8/1  "<VHAL_CANMsgInvalidBMS8_flg>"
  CANMsgInvalidBMS8/1 -> not6/1
  not6/1 -> bus_creator/6  "VINP_CANMsgValidBMS8_flg"
  bus_selector/7 -> CANMsgInvalidCCU1/1  "<VHAL_CANMsgInvalidCCU1_flg>"
  CANMsgInvalidCCU1/1 -> not7/1
  not7/1 -> bus_creator/7  "VINP_CANMsgValidCCU1_flg"
  bus_selector/8 -> CANMsgInvalidCCU2/1  "<VHAL_CANMsgInvalidCCU2_flg>"
  CANMsgInvalidCCU2/1 -> not8/1
  not8/1 -> bus_creator/8  "VINP_CANMsgValidCCU2_flg"
  bus_selector/9 -> CANMsgInvalidEBM1/1  "<VHAL_CANMsgInvalidEBM1_flg>"
  CANMsgInvalidEBM1/1 -> not9/1
  not9/1 -> bus_creator/9  "VINP_CANMsgValidEBM1_flg"
  bus_selector/10 -> CANMsgInvalidMCUBF1/1  "<VHAL_CANMsgInvalidMCUBF1_flg>"
  CANMsgInvalidMCUBF1/1 -> not10/1
  not10/1 -> bus_creator/10  "VINP_CANMsgValidMCUBF1_flg"
  bus_selector/11 -> CANMsgInvalidMCUBF2/1  "<VHAL_CANMsgInvalidMCUBF2_flg>"
  CANMsgInvalidMCUBF2/1 -> not11/1
  not11/1 -> bus_creator/11  "VINP_CANMsgValidMCUBF2_flg"
  bus_selector/12 -> CANMsgInvalidMCUBR1/1  "<VHAL_CANMsgInvalidMCUBR1_flg>"
  CANMsgInvalidMCUBR1/1 -> not12/1
  not12/1 -> bus_creator/12  "VINP_CANMsgValidMCUBR1_flg"
  bus_selector/13 -> CANMsgInvalidMCUBR2/1  "<VHAL_CANMsgInvalidMCUBR2_flg>"
  CANMsgInvalidMCUBR2/1 -> not13/1
  not13/1 -> bus_creator/13  "VINP_CANMsgValidMCUBR2_flg"
  bus_selector/14 -> CANMsgInvalidMCUNF1/1  "<VHAL_CANMsgInvalidMCUNF1_flg>"
  CANMsgInvalidMCUNF1/1 -> not14/1
  not14/1 -> bus_creator/14  "VINP_CANMsgValidMCUNF1_flg"
  bus_selector/15 -> CANMsgInvalidMCUNF2/1  "<VHAL_CANMsgInvalidMCUNF2_flg>"
  CANMsgInvalidMCUNF2/1 -> not15/1
  not15/1 -> bus_creator/15  "VINP_CANMsgValidMCUNF2_flg"
  bus_selector/16 -> CANMsgInvalidMCUNF3/1  "<VHAL_CANMsgInvalidMCUNF3_flg>"
  CANMsgInvalidMCUNF3/1 -> not16/1
  not16/1 -> bus_creator/16  "VINP_CANMsgValidMCUNF3_flg"
  bus_selector/17 -> CANMsgInvalidMCUNR1/1  "<VHAL_CANMsgInvalidMCUNR1_flg>"
  CANMsgInvalidMCUNR1/1 -> not17/1
  not17/1 -> bus_creator/17  "VINP_CANMsgValidMCUNR1_flg"
  bus_selector/18 -> CANMsgInvalidMCUNR2/1  "<VHAL_CANMsgInvalidMCUNR2_flg>"
  CANMsgInvalidMCUNR2/1 -> not18/1
  not18/1 -> bus_creator/18  "VINP_CANMsgValidMCUNR2_flg"
  bus_selector/19 -> CANMsgInvalidMCUNR3/1  "<VHAL_CANMsgInvalidMCUNR3_flg>"
  CANMsgInvalidMCUNR3/1 -> not19/1
  not19/1 -> bus_creator/19  "VINP_CANMsgValidMCUNR3_flg"
  bus_selector/20 -> CANMsgInvalidShifter1/1  "<VHAL_CANMsgInvalidShifter1_flg>"
  CANMsgInvalidShifter1/1 -> not20/1
  not20/1 -> bus_creator/20  "VINP_CANMsgValidShifter1_flg"
  bus_selector/21 -> CANMsgInvalidShifter2/1  "<VHAL_CANMsgInvalidShifter2_flg>"
  CANMsgInvalidShifter2/1 -> not21/1
  not21/1 -> bus_creator/21  "VINP_CANMsgValidShifter2_flg"
  [BHAL_outputs] -> bus_selector/1
  bus_creator/1 -> inp_CanValid_bus/1
